simulink model "tv_controller_final"  (R2024a)
settings: Solver=VariableStepAuto  StartTime=0.0  StopTime=10.0  RelTol=1e-3
values from neighbouring files (symbols this model uses):
  GCoSim_Name = 'GCoSim1'    [car_ver1_GCoSim1.m]    (also in car_ver1_GCoSim2.m = 'GCoSim2'; pure_GCoSim1.m)
  GCoSim_Name_n = r_temp___(2)    [car_ver1_GCoSim1.m]    (also in car_ver1_GCoSim2.m; pure_GCoSim1.m)
  Matlab_version = str2double(splited_Version__(1))    [car_ver1_GCoSim1.m]    (also in car_ver1_GCoSim2.m; pure_GCoSim1.m)
  Output_File = 'car_ver1_GCoSim1_GCoSim1'    [car_ver1_GCoSim1.m]    (also in car_ver1_GCoSim2.m = 'car_ver1_GCoSimulink_GCoSim2'; pure_GCoSim1.m = 'pure_GCoSim1')
  Output_file_n = r_temp___(2)    [car_ver1_GCoSim1.m]    (also in car_ver1_GCoSim2.m; pure_GCoSim1.m)
  Plant_inputs_num = r_temp___(1)    [car_ver1_GCoSim1.m]    (also in car_ver1_GCoSim2.m; pure_GCoSim1.m)
  Plant_outputs_num = r_temp___(1)    [car_ver1_GCoSim1.m]    (also in car_ver1_GCoSim2.m; pure_GCoSim1.m)
  RecurDyn = 'C:\Program Files\FunctionBay, Inc\RecurDyn 2024\Bin\'    [car_ver1_GCoSim1.m]    (also in car_ver1_GCoSim2.m; pure_GCoSim1.m)
  RecurDyn_controltimestep = 1.e-003    (= 0.001)    [car_ver1_GCoSim1.m]    (also in car_ver1_GCoSim2.m; pure_GCoSim1.m)
  RecurDyn_model = 'car_ver1.rdyn'    [car_ver1_GCoSim1.m]    (also in car_ver1_GCoSim2.m; pure_GCoSim1.m = 'pure.rdyn')
  RecurDyn_model_n = r_temp___(2)    [car_ver1_GCoSim1.m]    (also in car_ver1_GCoSim2.m; pure_GCoSim1.m)
libraries: simulink x1
settings Model: Creator=Dell  LastModifiedBy=Dell

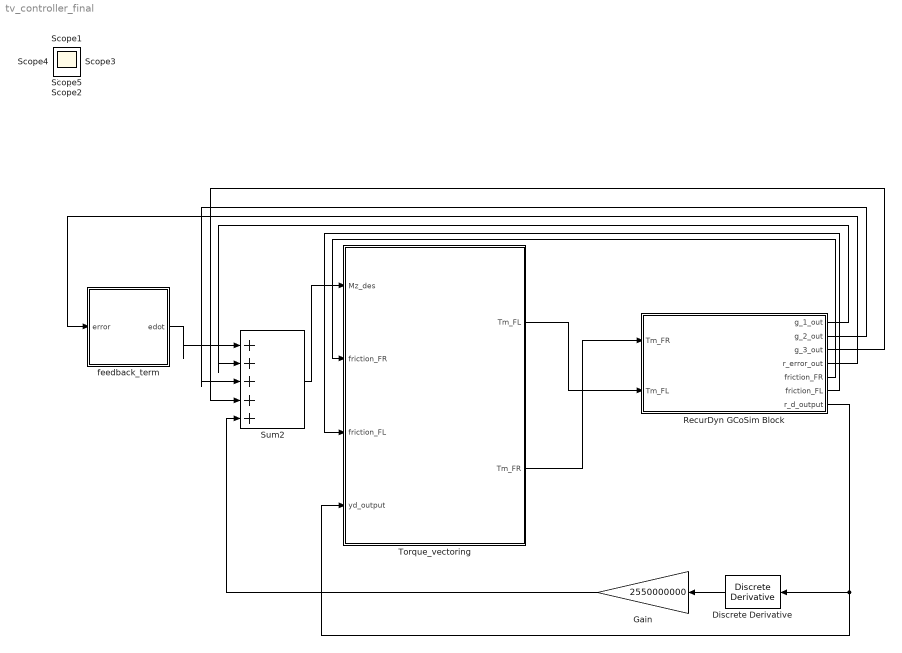
== system tv_controller_final ==
  Discrete Derivative : simulink/Discrete/Discrete Derivative  gainval=1.0  ICPrevScaledInput=0.0  OutMin=[]  OutMax=[]  OutDataType=fixdt(1, 16)  OutScaling=2^-10  DoSatur=off
  Gain : Gain  Gain=2550000000
  RecurDyn GCoSim Block : Subsystem
      mask Display: image(imread('RecurDyn_GCoSimIF_Host.png'))
  Sum2 : Sum  Inputs=|+++++
  Torque_vectoring : MATLAB Function  TreatAsAtomicUnit=on
  feedback_term : MATLAB Function  TreatAsAtomicUnit=on
  Scope{,1..5} (6 alike) : Scope
  wires:
  Sum2/1 -> Torque_vectoring/1(Mz_des)
  feedback_term/1(edot) -> Sum2/1
  Discrete Derivative/1 -> Gain/1
  Gain/1 -> Sum2/5
  Torque_vectoring/1(Tm_FL) -> RecurDyn GCoSim Block/2(Tm_FL)
  Torque_vectoring/2(Tm_FR) -> RecurDyn GCoSim Block/1(Tm_FR)
  RecurDyn GCoSim Block/5(friction_FR) -> Torque_vectoring/2(friction_FR)
  RecurDyn GCoSim Block/6(friction_FL) -> Torque_vectoring/3(friction_FL)
  RecurDyn GCoSim Block/7("r_d_output ") -> Discrete Derivative/1, Torque_vectoring/4(yd_output)
  RecurDyn GCoSim Block/4(r_error_out) -> feedback_term/1(error)
  RecurDyn GCoSim Block/2("g_2_out    ") -> Sum2/3
  RecurDyn GCoSim Block/3("g_3_out    ") -> Sum2/4
  RecurDyn GCoSim Block/1("g_1_out    ") -> Sum2/2

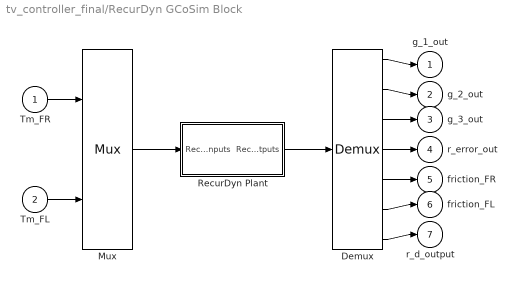
== system tv_controller_final/RecurDyn GCoSim Block ==
  Tm_FR : Inport
  Tm_FL : Inport  Port=2
  Demux : Demux  Outputs=7
      settings: DisplayOption=none
  Mux : Mux  Inputs=2
  RecurDyn Plant : Subsystem  mask(Recurdyn/Plant){RecurDyn_model_name=RecurDyn_model, GCoSim_Name_=GCoSim_Name, Output_File_Name_=Output_File, RecurDyn_=RecurDyn, Matlab_version_=Matlab_version, RecurDyn_controltimestep_=RecurDyn_controltimestep, RecurDyn_step_=100, Waitingtime=1000, RecurDyn_static_=off, RecurDyn_show_=on, RecurDyn_ani_=on, Create_Output_Folder_=off}
      mask prompts: GCoSim_Name_ "GCoSim Name"; Output_File_Name_ "Output File Name"; RecurDyn_ "RecurDyn_install_directory"; Matlab_version_ "Matlab version"; RecurDyn_controltimestep_ "Sampling period"; RecurDyn_step_ "RecurDyn_step"; Waitingtime "Waiting time"; RecurDyn_static_ "Static analysis"; RecurDyn_show_ "RecurDyn_show"; RecurDyn_ani_ "RecurDyn_animation"; Create_Output_Folder_ "Create Output Folder"
      mask help:
      | This block is able to simulate for any Recurdyn Dynamics Model as Recurdyn/GCoSim Solver.
      | All Data of Plant inputs/outputs are transfered at every sampling time which is defined by Sampling Period (Control Time Step).
      mask Display: disp( 'Dynamic Model' )
  "g_1_out    " : Outport
  "g_2_out    " : Outport  Port=2
  "g_3_out    " : Outport  Port=3
  r_error_out : Outport  Port=4
  friction_FR : Outport  Port=5
  friction_FL : Outport  Port=6
  "r_d_output " : Outport  Port=7
  wires:
  RecurDyn Plant/1(RecurDyn_outputs) -> Demux/1
  Mux/1 -> RecurDyn Plant/1(" RecurDyn_inputs")
  Demux/1 -> "g_1_out    "/1
  Demux/2 -> "g_2_out    "/1
  Demux/3 -> "g_3_out    "/1
  Demux/4 -> r_error_out/1
  Demux/5 -> friction_FR/1
  Demux/6 -> friction_FL/1
  Demux/7 -> "r_d_output "/1
  Tm_FR/1 -> Mux/1
  Tm_FL/1 -> Mux/2

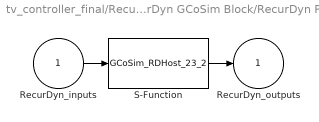
== system tv_controller_final/RecurDyn GCoSim Block/RecurDyn Plant ==
  " RecurDyn_inputs" : Inport
  S-Function : S-Function  FunctionName=GCoSim_RDHost_23_2  Parameters=RecurDyn_controltimestep_,RecurDyn_model_name,RecurDyn_,RecurDyn_static_,RecurDyn_step_,RecurDyn_show_,RecurDyn_ani_,Matlab_version_,RecurDyn_model_n,Plant_inputs_num,Plant_outputs_num,Waitingtime,Create_Output_Folder_,Output_File_Name_,Output_file_n,GCoSim_Name_,GCoSim_Name_n  SFunctionDeploymentMode=off  EnableBusSupport=off
  RecurDyn_outputs : Outport  InitialOutput=0  VectorParamsAs1DForOutWhenUnconnected=off
  wires:
  S-Function/1 -> RecurDyn_outputs/1
  " RecurDyn_inputs"/1 -> S-Function/1

== matlab function tv_controller_final/feedback_term ==
  data: error input; edot output
function edot = sat_e (error)

positive_proportional_gain = 0.62;
pos_sat_boundary = 0.7; %이부분 정확하게
Iz = 2550000000;
if pos_sat_boundary<error
    sat_e = 1;
elseif error < -pos_sat_boundary
    sat_e = -1;
else
    sat_e = error / pos_sat_boundary;
end

edot = - Iz *positive_proportional_gain * sat_e;
%edot = - positive_proportional_gain * sat_e;

== matlab function tv_controller_final/Torque_vectoring ==
  data: Tm_FL output; Mz_des input; Tm_FR output; friction_FR input; friction_FL input; yd_output input
function [ Tm_FL, Tm_FR ] = Torque_distribution (Mz_des ,friction_FR, friction_FL , yd_output )
m = 1500; % kg
g = 9810; % mm/s^2
L = 2746.83;
Lf = 900;
Lr = 1846.83;
h = 300; % height of CG, mm
t = 1600; %track width
Re = 300; % Effective tire radius, mm
Cf = 50000; %N/rad 실제 차아님 논문참
Cr = 50000;
%vx = vx * 277.83;
%vy = vy * 277.83;
Mz_des = Mz_des / 1e3
Tm_reg_m = 1000000;
if Mz_des >= 0 
    Mz_lim = t*(friction_FR - Tm_reg_m) / (2*Re);
else
    Mz_lim = t*(friction_FL - Tm_reg_m) / (2*Re);
end
%계산된 최대 모멘트, desired 모멘트로 토크 분배
alpha = 0.62; %(0<=alpha<=1),  By adjusting 𝛼, it is possible to freely tune the timing of the negative IWM torque intervention

Mz_des
Mz_lim_alpha = alpha*Mz_lim


if Mz_des < -Mz_lim_alpha
   Tm_FL = Re*(alpha*Mz_lim - Mz_des) / t;
    disp('A')
elseif Mz_des <0
    Tm_FL = -Re*Mz_des / t; %여기 Mz_des_f라 되있는데 오탄가..?
    disp('B')   
elseif Mz_des <=Mz_lim_alpha
    Tm_FL = 0;
    disp('C')    
else
    Tm_FL = Re*(alpha * Mz_lim - Mz_des) / t;    
    disp('D')
end


if Mz_des < -Mz_lim_alpha
    Tm_FR = Re*(alpha*Mz_lim + Mz_des) / t;
elseif Mz_des <0
    Tm_FR = 0;
elseif Mz_des <=Mz_lim_alpha
    Tm_FR = Re*Mz_des / t;
else
    Tm_FR = Re*(alpha * Mz_lim + Mz_des) / t;
end
Tm_FL = Tm_FL / 1e1
Tm_FR = Tm_FR / 1e1

yd_output
